simulink model "ES228A_HwTqArbn"
settings: Solver=ode45  StartTime=0.0  StopTime=10.0  RelTol=1e-3
values from neighbouring files (symbols this model uses):
  HWTQSCA_CNT_U08 = DataDict.Constant    [ES228A_HwTqArbn_DataDict.m]
libraries: simulink x9, NexteerUtilities x3
settings DataIOCC: LimitDataPoints=on  SaveFormat=Array  ReturnWorkspaceOutputs=off
settings OptimizationCC: LifeSpan=inf  SimCompilerOptimization=Off
settings DebuggingCC: UnderspecifiedInitializationDetection=Classic  MergeDetectMultiDrivingBlocksExec=none  SolverPrmCheckMsg=warning  FcnCallInpInsideContextMsg=EnableAllAsError  FrameProcessingCompatibilityMsg=warning  SFUnexpectedBacktrackingDiag=warning  SFNoUnconditionalDefaultTransitionDiag=warning
settings HardwareCC: ProdBitPerPointer=32  ProdLargestAtomicFloat=None  ProdIntDivRoundTo=Undefined  ProdEndianess=Unspecified  ProdWordSize=32  ProdHWDeviceType=32-bit Generic
settings ModelReferenceCC: PropagateSignalLabelsOutOfModel=off
settings SFSimCC: SimUseLocalCustomCode=off
settings RTWCC: RTWUseLocalCustomCode=off  RTWCompilerOptimization=Off
settings GRTTargetCC: CodeReplacementLibrary=ANSI_C  GeneratePreprocessorConditionals=Disable all  CPPClassGenCompliant=off

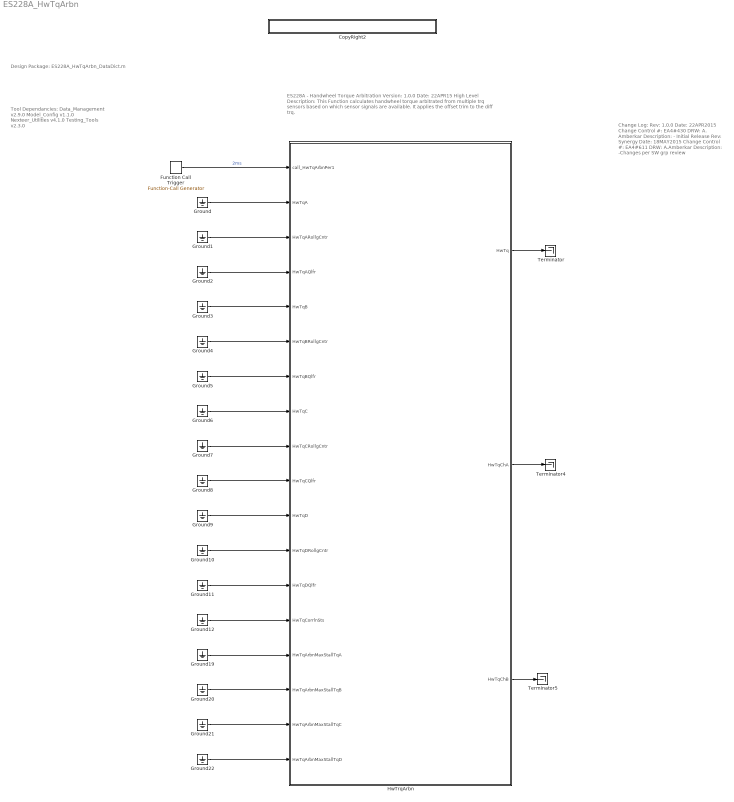
== system ES228A_HwTqArbn ==
  note: Design Package:
      |
      | ES228A_HwTqArbn_DataDict.m
  note: Tool Dependancies:
      |
      | Data_Management v2.9.0
      | Model_Config v1.1.0
      | Nexteer_Utilities v4.1.0
      | Testing_Tools v2.3.0
  note: Change Log:
      |
      | Rev: 1.0.0
      | Date: 22APR2015
      | Change Control #: EA4#430
      | DRW: A. Amberkar
      | Description:
      | - Initial Release
      |
      | Rev: Synergy
      | Date: 18MAY2015
      | Change Control #: EA4#611
      | DRW: A.Amberkar
      | Description:
      | -Changes per SW grp review
  note: ES228A - Handwheel Torque Arbitration
      |
      | Version: 1.0.0
      | Date: 22APR15
      |
      | High Level Description:
      | This Function calculates handwheel torque arbitrated from multiple trq sensors based
      | on which sensor signals are available.  It applies the offset trim to the diff trq.
  CopyRight2 : Subsystem  Description=|  mask(Copyright Information){none=on}
      | Copyright info block.                                               
      |                                                                     
      | Place copyright information at the top of every subsystem in design.
      mask prompts: none "No parameters"
      mask help: Place copyright information at the top of every subsystem in design.
      mask Display:
      | NxtrConf = 'Nexteer Confidential';
      | 
      | sys = bdroot; %handle for the current model ("system")
      | first = get_param(sys,'Created');
      | first = first(end-3:end);  %year is last four digits
      | 
      | last = get_param(sys,'LastModifiedDate');
      | if isempty(last)
      |     last = datestr(now,'yyyy');
      | else
      |     last = last(end-3:end);
      | end
      | 
      | if strcmp(first,last)
      |     fprintf('%s -- Copyright %s Nexteer',NxtrConf,first)
      | else
      |     fprintf('%s -- %s%s- %s Nexteer',NxtrConf,char(169),first,last)
      | end
  Function Call Trigger : simulink/Ports & Subsystems/Function-Call Generator  sample_time=.002  numberOfIterations=1
  Ground{,1..12,19..22} (17 alike) : Ground
  HwTrqArbn : Subsystem
  Terminator : Terminator
  Terminator4 : Terminator
  Terminator5 : Terminator
  wires:
  Function Call Trigger/1 -> HwTrqArbn/1(call_HwTqArbnPer1)  "2ms"
  HwTrqArbn/2(HwTqChA) -> Terminator4/1
  HwTrqArbn/1(HwTq) -> Terminator/1
  Ground1/1 -> HwTrqArbn/3(HwTqARollgCntr)
  Ground3/1 -> HwTrqArbn/5(HwTqB)
  Ground5/1 -> HwTrqArbn/7(HwTqBQlfr)
  Ground9/1 -> HwTrqArbn/11(HwTqD)
  Ground10/1 -> HwTrqArbn/12(HwTqDRollgCntr)
  Ground11/1 -> HwTrqArbn/13(HwTqDQlfr)
  Ground12/1 -> HwTrqArbn/14(HwTqCorrlnSts)
  Ground20/1 -> HwTrqArbn/16(HwTqArbnMaxStallTqB)
  Ground21/1 -> HwTrqArbn/17(HwTqArbnMaxStallTqC)
  Ground22/1 -> HwTrqArbn/18(HwTqArbnMaxStallTqD)
  Ground8/1 -> HwTrqArbn/10(HwTqCQlfr)
  Ground4/1 -> HwTrqArbn/6(HwTqBRollgCntr)
  Ground/1 -> HwTrqArbn/2(HwTqA)
  HwTrqArbn/3(HwTqChB) -> Terminator5/1
  Ground2/1 -> HwTrqArbn/4(HwTqAQlfr)
  Ground19/1 -> HwTrqArbn/15("HwTqArbnMaxStallTqA ")
  Ground7/1 -> HwTrqArbn/9(HwTqCRollgCntr)
  Ground6/1 -> HwTrqArbn/8(HwTqC)

== system ES228A_HwTqArbn/CopyRight2 ==

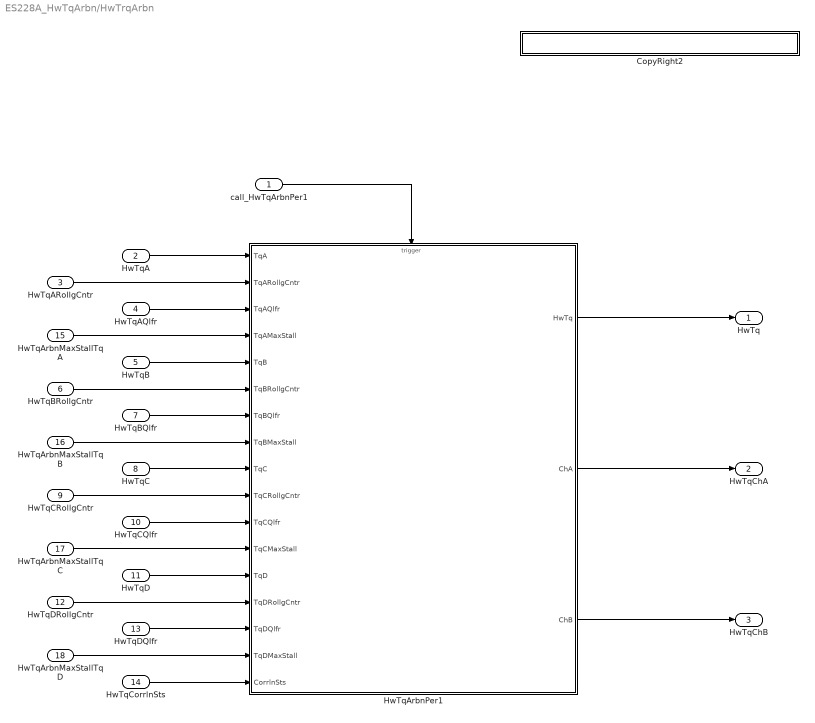
== system ES228A_HwTqArbn/HwTrqArbn ==
  call_HwTqArbnPer1 : Inport
  HwTqA : Inport  Port=2
  HwTqARollgCntr : Inport  Port=3
  HwTqAQlfr : Inport  Port=4
  HwTqB : Inport  Port=5
  HwTqBRollgCntr : Inport  Port=6
  HwTqBQlfr : Inport  Port=7
  HwTqC : Inport  Port=8
  HwTqCRollgCntr : Inport  Port=9
  HwTqCQlfr : Inport  Port=10
  HwTqD : Inport  Port=11
  HwTqDRollgCntr : Inport  Port=12
  HwTqDQlfr : Inport  Port=13
  HwTqCorrlnSts : Inport  Port=14
  "HwTqArbnMaxStallTqA " : Inport  Port=15
  HwTqArbnMaxStallTqB : Inport  Port=16
  HwTqArbnMaxStallTqC : Inport  Port=17
  HwTqArbnMaxStallTqD : Inport  Port=18
  CopyRight2 : Subsystem  Description=|  mask(Copyright Information){none=on}
      | Copyright info block.                                               
      |                                                                     
      | Place copyright information at the top of every subsystem in design.
      mask prompts: none "No parameters"
      mask help: Place copyright information at the top of every subsystem in design.
      mask Display:
      | NxtrConf = 'Nexteer Confidential';
      | 
      | sys = bdroot; %handle for the current model ("system")
      | first = get_param(sys,'Created');
      | first = first(end-3:end);  %year is last four digits
      | 
      | last = get_param(sys,'LastModifiedDate');
      | if isempty(last)
      |     last = datestr(now,'yyyy');
      | else
      |     last = last(end-3:end);
      | end
      | 
      | if strcmp(first,last)
      |     fprintf('%s -- Copyright %s Nexteer',NxtrConf,first)
      | else
      |     fprintf('%s -- %s%s- %s Nexteer',NxtrConf,char(169),first,last)
      | end
  HwTqArbnPer1 : Subsystem  RequirementInfo="{'linktype_rmi_doors' '0000c476 (/ESG Group/FDD Module Requirements/EA4 Specific/ES228A_HwTqArbn)' '#ES228A_85' 'true' 'REQ:  ES228A_85' '' } %GIDa_343f2210_b87e_41f4_8880_c295a6f80a3f"  TreatAsAtomicUnit=on
  HwTq : Outport
  HwTqChA : Outport  Port=2
  HwTqChB : Outport  Port=3
  wires:
  call_HwTqArbnPer1/1 -> HwTqArbnPer1/Trigger
  HwTqARollgCntr/1 -> HwTqArbnPer1/2(TqARollgCntr)
  HwTqAQlfr/1 -> HwTqArbnPer1/3(TqAQlfr)
  HwTqBRollgCntr/1 -> HwTqArbnPer1/6(TqBRollgCntr)
  HwTqBQlfr/1 -> HwTqArbnPer1/7(TqBQlfr)
  HwTqCRollgCntr/1 -> HwTqArbnPer1/10(TqCRollgCntr)
  HwTqCQlfr/1 -> HwTqArbnPer1/11(TqCQlfr)
  HwTqDRollgCntr/1 -> HwTqArbnPer1/14(TqDRollgCntr)
  HwTqDQlfr/1 -> HwTqArbnPer1/15(TqDQlfr)
  "HwTqArbnMaxStallTqA "/1 -> HwTqArbnPer1/4(TqAMaxStall)
  HwTqCorrlnSts/1 -> HwTqArbnPer1/17(CorrlnSts)
  HwTqArbnMaxStallTqC/1 -> HwTqArbnPer1/12(TqCMaxStall)
  HwTqArbnMaxStallTqD/1 -> HwTqArbnPer1/16(TqDMaxStall)
  HwTqA/1 -> HwTqArbnPer1/1(TqA)
  HwTqB/1 -> HwTqArbnPer1/5(TqB)
  HwTqArbnMaxStallTqB/1 -> HwTqArbnPer1/8(TqBMaxStall)
  HwTqC/1 -> HwTqArbnPer1/9(TqC)
  HwTqD/1 -> HwTqArbnPer1/13(TqD)
  HwTqArbnPer1/1(HwTq) -> HwTq/1
  HwTqArbnPer1/2(ChA) -> HwTqChA/1
  HwTqArbnPer1/3(ChB) -> HwTqChB/1

== system ES228A_HwTqArbn/HwTrqArbn/CopyRight2 ==

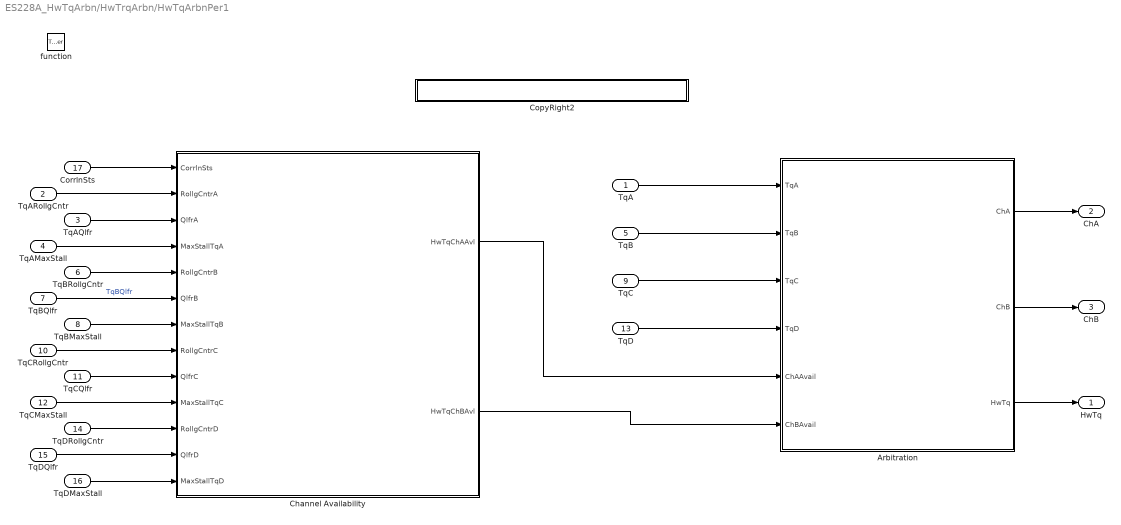
== system ES228A_HwTqArbn/HwTrqArbn/HwTqArbnPer1 ==
  TqA : Inport
  TqARollgCntr : Inport  Port=2
  TqAQlfr : Inport  Port=3
  TqAMaxStall : Inport  Port=4
  TqB : Inport  Port=5
  TqBRollgCntr : Inport  Port=6
  TqBQlfr : Inport  Port=7
  TqBMaxStall : Inport  Port=8
  TqC : Inport  Port=9
  TqCRollgCntr : Inport  Port=10
  TqCQlfr : Inport  Port=11
  TqCMaxStall : Inport  Port=12
  TqD : Inport  Port=13
  TqDRollgCntr : Inport  Port=14
  TqDQlfr : Inport  Port=15
  TqDMaxStall : Inport  Port=16
  CorrlnSts : Inport  Port=17
  function : TriggerPort  TriggerType=function-call
  Arbitration : Subsystem  RequirementInfo="{'linktype_rmi_doors' '0000c476 (/ESG Group/FDD Module Requirements/EA4 Specific/ES228A_HwTqArbn)' '#ES228A_128' 'true' 'REQ:  ES228A_128' '' ; 'linktype_rmi_doors' '0000c476 (/ESG Group/FDD Module Requirements/EA4 Specific/ES228A_HwTqArbn)' '#ES228A_98' 'true' 'REQ:  ES228A_98' '' } %GIDa_5e475dce_6d1a_4377_b1f7_ac9d58e1cf5d"
  Channel Availability : Subsystem
  CopyRight2 : Subsystem  Description=|  mask(Copyright Information){none=on}
      | Copyright info block.                                               
      |                                                                     
      | Place copyright information at the top of every subsystem in design.
      mask prompts: none "No parameters"
      mask help: Place copyright information at the top of every subsystem in design.
      mask Display:
      | NxtrConf = 'Nexteer Confidential';
      | 
      | sys = bdroot; %handle for the current model ("system")
      | first = get_param(sys,'Created');
      | first = first(end-3:end);  %year is last four digits
      | 
      | last = get_param(sys,'LastModifiedDate');
      | if isempty(last)
      |     last = datestr(now,'yyyy');
      | else
      |     last = last(end-3:end);
      | end
      | 
      | if strcmp(first,last)
      |     fprintf('%s -- Copyright %s Nexteer',NxtrConf,first)
      | else
      |     fprintf('%s -- %s%s- %s Nexteer',NxtrConf,char(169),first,last)
      | end
  HwTq : Outport
  ChA : Outport  Port=2
  ChB : Outport  Port=3
  wires:
  CorrlnSts/1 -> Channel Availability/1(CorrlnSts)
  TqAQlfr/1 -> Channel Availability/3(QlfrA)
  TqAMaxStall/1 -> Channel Availability/4(MaxStallTqA)
  TqBRollgCntr/1 -> Channel Availability/5(RollgCntrB)
  TqBQlfr/1 -> Channel Availability/6(QlfrB)  "TqBQlfr"
  TqBMaxStall/1 -> Channel Availability/7(MaxStallTqB)
  TqCRollgCntr/1 -> Channel Availability/8(RollgCntrC)
  TqCQlfr/1 -> Channel Availability/9(QlfrC)
  TqCMaxStall/1 -> Channel Availability/10(MaxStallTqC)
  TqDRollgCntr/1 -> Channel Availability/11(RollgCntrD)
  TqDQlfr/1 -> Channel Availability/12(QlfrD)
  TqDMaxStall/1 -> Channel Availability/13(MaxStallTqD)
  TqARollgCntr/1 -> Channel Availability/2(RollgCntrA)
  TqA/1 -> Arbitration/1(TqA)
  TqB/1 -> Arbitration/2(TqB)
  TqC/1 -> Arbitration/3(TqC)
  TqD/1 -> Arbitration/4(TqD)
  Channel Availability/1(HwTqChAAvl) -> Arbitration/5(ChAAvail)
  Channel Availability/2(HwTqChBAvl) -> Arbitration/6(ChBAvail)
  Arbitration/3(HwTq) -> HwTq/1
  Arbitration/2(ChB) -> ChB/1
  Arbitration/1(ChA) -> ChA/1

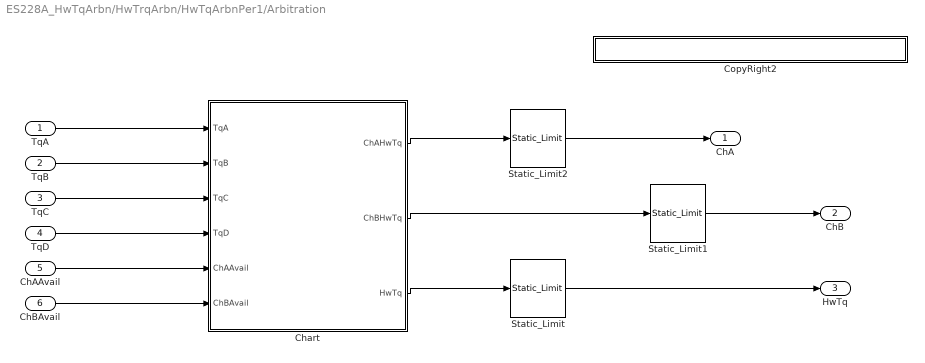
== system ES228A_HwTqArbn/HwTrqArbn/HwTqArbnPer1/Arbitration ==
  TqA : Inport
  TqB : Inport  Port=2
  TqC : Inport  Port=3
  TqD : Inport  Port=4
  ChAAvail : Inport  Port=5
  ChBAvail : Inport  Port=6
  Chart : Stateflow chart  RequirementInfo="{'linktype_rmi_doors' '0000c476 (/ESG Group/FDD Module Requirements/EA4 Specific/ES228A_HwTqArbn)' '#ES228A_83' 'true' 'REQ:  ES228A_83' '' } %GIDa_6d64dbbd_6a35_4759_a8d5_33867a77d9f5"  TreatAsAtomicUnit=on
  CopyRight2 : Subsystem  Description=|  mask(Copyright Information){none=on}
      | Copyright info block.                                               
      |                                                                     
      | Place copyright information at the top of every subsystem in design.
      mask prompts: none "No parameters"
      mask help: Place copyright information at the top of every subsystem in design.
      mask Display:
      | NxtrConf = 'Nexteer Confidential';
      | 
      | sys = bdroot; %handle for the current model ("system")
      | first = get_param(sys,'Created');
      | first = first(end-3:end);  %year is last four digits
      | 
      | last = get_param(sys,'LastModifiedDate');
      | if isempty(last)
      |     last = datestr(now,'yyyy');
      | else
      |     last = last(end-3:end);
      | end
      | 
      | if strcmp(first,last)
      |     fprintf('%s -- Copyright %s Nexteer',NxtrConf,first)
      | else
      |     fprintf('%s -- %s%s- %s Nexteer',NxtrConf,char(169),first,last)
      | end
  Static_Limit : NexteerUtilities/Static_Limit  uprlim=HWTQMAXLIM_HWNWTMTR_F32  lwrlim=HWTQMINLIM_HWNWTMTR_F32
      settings: AttributesFormatString=|
      | Upper Limit:%<uprlim>
      | Lower Limit:%<lwrlim>
  Static_Limit1 : NexteerUtilities/Static_Limit  uprlim=HWTQMAXLIM_HWNWTMTR_F32  lwrlim=HWTQMINLIM_HWNWTMTR_F32
      settings: AttributesFormatString=|
      | Upper Limit:%<uprlim>
      | Lower Limit:%<lwrlim>
  Static_Limit2 : NexteerUtilities/Static_Limit  uprlim=HWTQMAXLIM_HWNWTMTR_F32  lwrlim=HWTQMINLIM_HWNWTMTR_F32
      settings: AttributesFormatString=|
      | Upper Limit:%<uprlim>
      | Lower Limit:%<lwrlim>
  ChA : Outport
  ChB : Outport  Port=2
  HwTq : Outport  Port=3
  wires:
  TqA/1 -> Chart/1(TqA)
  TqB/1 -> Chart/2(TqB)
  TqC/1 -> Chart/3(TqC)
  TqD/1 -> Chart/4(TqD)
  ChAAvail/1 -> Chart/5(ChAAvail)
  ChBAvail/1 -> Chart/6(ChBAvail)
  Chart/1(ChAHwTq) -> Static_Limit2/1
  Chart/2(ChBHwTq) -> Static_Limit1/1
  Chart/3(HwTq) -> Static_Limit/1
  Static_Limit/1 -> HwTq/1
  Static_Limit1/1 -> ChB/1
  Static_Limit2/1 -> ChA/1

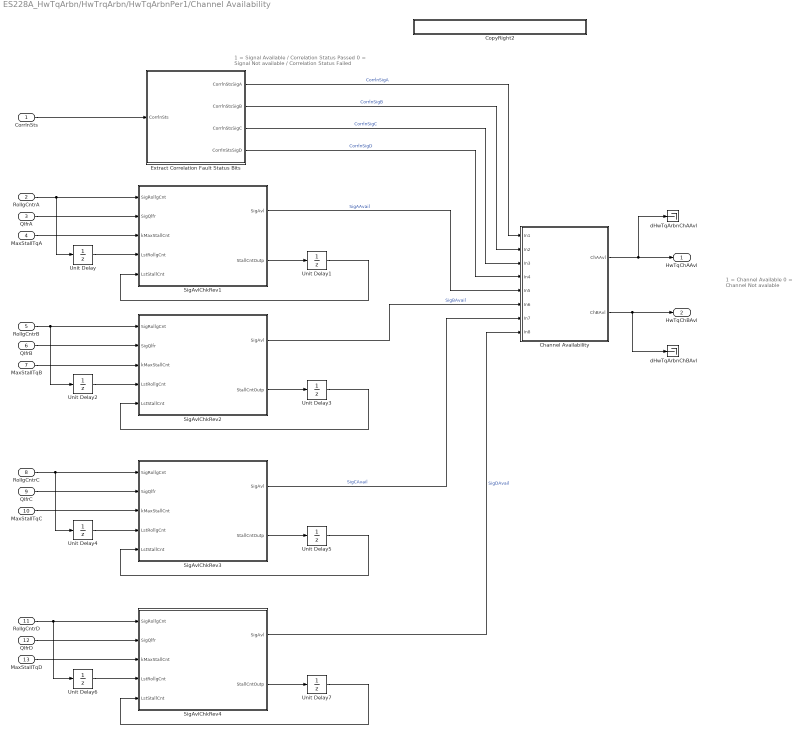
== system ES228A_HwTqArbn/HwTrqArbn/HwTqArbnPer1/Channel Availability ==
  note: 1 = Channel Available
      | 0 = Channel Not avalable
  note: 1 = Signal Available / Correlation Status Passed
      | 0 = Signal Not available / Correlation Status Failed
  CorrlnSts : Inport
  RollgCntrA : Inport  Port=2
  QlfrA : Inport  Port=3
  MaxStallTqA : Inport  Port=4
  RollgCntrB : Inport  Port=5
  QlfrB : Inport  Port=6
  MaxStallTqB : Inport  Port=7
  RollgCntrC : Inport  Port=8
  QlfrC : Inport  Port=9
  MaxStallTqC : Inport  Port=10
  RollgCntrD : Inport  Port=11
  QlfrD : Inport  Port=12
  MaxStallTqD : Inport  Port=13
  Channel Availability : Subsystem  RequirementInfo="{'linktype_rmi_doors' '0000c476 (/ESG Group/FDD Module Requirements/EA4 Specific/ES228A_HwTqArbn)' '#ES228A_129' 'true' 'REQ:  ES228A_129' '' ; 'linktype_rmi_doors' '0000c476 (/ESG Group/FDD Module Requirements/EA4 Specific/ES228A_HwTqArbn)' '#ES228A_91' 'true' 'REQ:  ES228A_91' '' } %GIDa_746ca483_b495_4e00_a250_9b34cc012507"
  CopyRight2 : Subsystem  Description=|  mask(Copyright Information){none=on}
      | Copyright info block.                                               
      |                                                                     
      | Place copyright information at the top of every subsystem in design.
      mask prompts: none "No parameters"
      mask help: Place copyright information at the top of every subsystem in design.
      mask Display:
      | NxtrConf = 'Nexteer Confidential';
      | 
      | sys = bdroot; %handle for the current model ("system")
      | first = get_param(sys,'Created');
      | first = first(end-3:end);  %year is last four digits
      | 
      | last = get_param(sys,'LastModifiedDate');
      | if isempty(last)
      |     last = datestr(now,'yyyy');
      | else
      |     last = last(end-3:end);
      | end
      | 
      | if strcmp(first,last)
      |     fprintf('%s -- Copyright %s Nexteer',NxtrConf,first)
      | else
      |     fprintf('%s -- %s%s- %s Nexteer',NxtrConf,char(169),first,last)
      | end
  Extract Correlation Fault Status Bits : Subsystem  RequirementInfo="{'linktype_rmi_doors' '0000c476 (/ESG Group/FDD Module Requirements/EA4 Specific/ES228A_HwTqArbn)' '#ES228A_129' 'true' 'REQ:  ES228A_129' '' } %GIDa_e59e4d92_3888_4f3c_9500_97095e00bcfc"
  SigAvlChkRev1 : Stateflow chart  RequirementInfo="{'linktype_rmi_doors' '0000c476 (/ESG Group/FDD Module Requirements/EA4 Specific/ES228A_HwTqArbn)' '#ES228A_91' 'true' 'REQ:  ES228A_91' '' } %GIDa_e4c178c2_f8a5_42cf_ac9f_6f496b5237f8"  TreatAsAtomicUnit=on
  SigAvlChkRev2 : Stateflow chart  RequirementInfo="{'linktype_rmi_doors' '0000c476 (/ESG Group/FDD Module Requirements/EA4 Specific/ES228A_HwTqArbn)' '#ES228A_91' 'true' 'REQ:  ES228A_91' '' } %GIDa_b0676f02_3d97_45d5_aa8a_49c82560c074"  TreatAsAtomicUnit=on
  SigAvlChkRev3 : Stateflow chart  RequirementInfo="{'linktype_rmi_doors' '0000c476 (/ESG Group/FDD Module Requirements/EA4 Specific/ES228A_HwTqArbn)' '#ES228A_91' 'true' 'REQ:  ES228A_91' '' } %GIDa_99c29bb1_dae8_491f_835b_8ea19b5dfde5"  TreatAsAtomicUnit=on
  SigAvlChkRev4 : Stateflow chart  RequirementInfo="{'linktype_rmi_doors' '0000c476 (/ESG Group/FDD Module Requirements/EA4 Specific/ES228A_HwTqArbn)' '#ES228A_91' 'true' 'REQ:  ES228A_91' '' } %GIDa_0917a9fe_5043_4981_abf9_3e4589195506"  TreatAsAtomicUnit=on
  Unit Delay : UnitDelay  SampleTime=-1  StateName=HwTqArbnTqARollgCntrPrev  StateMustResolveToSignalObject=on
      settings: AttributesFormatString=|
      | State Variable:
      | %<StateName>
  Unit Delay1 : UnitDelay  SampleTime=-1  StateName=HwTqArbnTqAStallCntrPrev  StateMustResolveToSignalObject=on
      settings: AttributesFormatString=|
      | State Variable:
      | %<StateName>
  Unit Delay2 : UnitDelay  SampleTime=-1  StateName=HwTqArbnTqBRollgCntrPrev  StateMustResolveToSignalObject=on
      settings: AttributesFormatString=|
      | State Variable:
      | %<StateName>
  Unit Delay3 : UnitDelay  SampleTime=-1  StateName=HwTqArbnTqBStallCntrPrev  StateMustResolveToSignalObject=on
      settings: AttributesFormatString=|
      | State Variable:
      | %<StateName>
  Unit Delay4 : UnitDelay  SampleTime=-1  StateName=HwTqArbnTqCRollgCntrPrev  StateMustResolveToSignalObject=on
      settings: AttributesFormatString=|
      | State Variable:
      | %<StateName>
  Unit Delay5 : UnitDelay  SampleTime=-1  StateName=HwTqArbnTqCStallCntrPrev  StateMustResolveToSignalObject=on
      settings: AttributesFormatString=|
      | State Variable:
      | %<StateName>
  Unit Delay6 : UnitDelay  SampleTime=-1  StateName=HwTqArbnTqDRollgCntrPrev  StateMustResolveToSignalObject=on
      settings: AttributesFormatString=|
      | State Variable:
      | %<StateName>
  Unit Delay7 : UnitDelay  SampleTime=-1  StateName=HwTqArbnTqDStallCntrPrev  StateMustResolveToSignalObject=on
      settings: AttributesFormatString=|
      | State Variable:
      | %<StateName>
  "dHwTqArbnChAAvl " : Terminator
  "dHwTqArbnChBAvl " : Terminator
  HwTqChAAvl : Outport
  HwTqChBAvl : Outport  Port=2
  wires:
  CorrlnSts/1 -> Extract Correlation Fault Status Bits/1(CorrlnSts)
  Extract Correlation Fault Status Bits/1(CorrlnStsSigA) -> Channel Availability/1(In1)  "CorrlnSigA"
  Extract Correlation Fault Status Bits/2(CorrlnStsSigB) -> Channel Availability/2(In2)  "CorrlnSigB"
  Extract Correlation Fault Status Bits/3(CorrlnStsSigC) -> Channel Availability/3(In3)  "CorrlnSigC"
  Extract Correlation Fault Status Bits/4(CorrlnStsSigD) -> Channel Availability/4(In4)  "CorrlnSigD"
  SigAvlChkRev1/1(SigAvl) -> Channel Availability/5(In5)  "SigAAvail"
  SigAvlChkRev2/1(SigAvl) -> Channel Availability/6(In6)  "SigBAvail"
  SigAvlChkRev3/1(SigAvl) -> Channel Availability/7(In7)  "SigCAvail"
  SigAvlChkRev4/1(SigAvl) -> Channel Availability/8(In8)  "SigDAvail"
  Channel Availability/1(ChAAvl) -> "dHwTqArbnChAAvl "/1, HwTqChAAvl/1
  Channel Availability/2(ChBAvl) -> "dHwTqArbnChBAvl "/1, HwTqChBAvl/1
  RollgCntrA/1 -> Unit Delay/1, SigAvlChkRev1/1(SigRollgCnt)
  QlfrA/1 -> SigAvlChkRev1/2(SigQlfr)
  MaxStallTqA/1 -> SigAvlChkRev1/3(kMaxStallCnt)
  RollgCntrB/1 -> Unit Delay2/1, SigAvlChkRev2/1(SigRollgCnt)
  QlfrB/1 -> SigAvlChkRev2/2(SigQlfr)
  MaxStallTqB/1 -> SigAvlChkRev2/3(kMaxStallCnt)
  RollgCntrC/1 -> Unit Delay4/1, SigAvlChkRev3/1(SigRollgCnt)
  QlfrC/1 -> SigAvlChkRev3/2(SigQlfr)
  MaxStallTqC/1 -> SigAvlChkRev3/3(kMaxStallCnt)
  RollgCntrD/1 -> Unit Delay6/1, SigAvlChkRev4/1(SigRollgCnt)
  QlfrD/1 -> SigAvlChkRev4/2(SigQlfr)
  MaxStallTqD/1 -> SigAvlChkRev4/3(kMaxStallCnt)
  Unit Delay/1 -> SigAvlChkRev1/4(LstRollgCnt)
  SigAvlChkRev1/2(StallCntOutp) -> Unit Delay1/1
  Unit Delay1/1 -> SigAvlChkRev1/5(LstStallCnt)
  Unit Delay2/1 -> SigAvlChkRev2/4(LstRollgCnt)
  SigAvlChkRev2/2(StallCntOutp) -> Unit Delay3/1
  Unit Delay3/1 -> SigAvlChkRev2/5(LstStallCnt)
  Unit Delay4/1 -> SigAvlChkRev3/4(LstRollgCnt)
  SigAvlChkRev3/2(StallCntOutp) -> Unit Delay5/1
  Unit Delay5/1 -> SigAvlChkRev3/5(LstStallCnt)
  Unit Delay6/1 -> SigAvlChkRev4/4(LstRollgCnt)
  SigAvlChkRev4/2(StallCntOutp) -> Unit Delay7/1
  Unit Delay7/1 -> SigAvlChkRev4/5(LstStallCnt)

== system ES228A_HwTqArbn/HwTrqArbn/HwTqArbnPer1/CopyRight2 ==

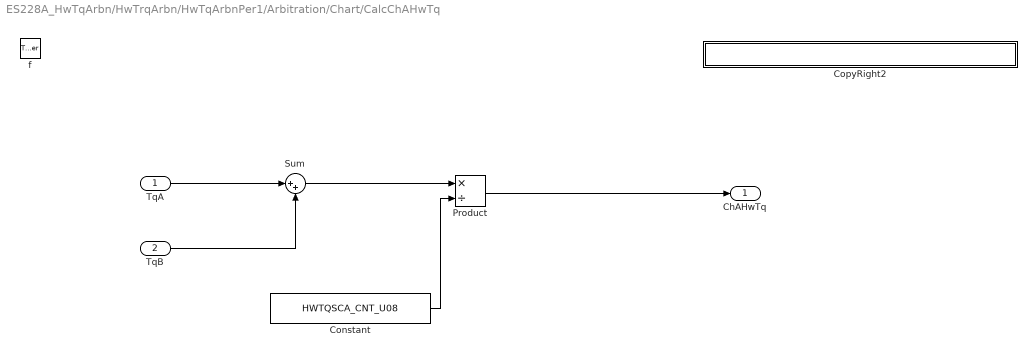
== system ES228A_HwTqArbn/HwTrqArbn/HwTqArbnPer1/Arbitration/Chart/CalcChAHwTq ==
  TqA : Inport
  TqB : Inport  Port=2
  f : TriggerPort  TriggerType=function-call
      settings: CopyFcn=Stateflow.SLINSF.SimulinkMan.removeBlockPreDeleteFcn  PreDeleteFcn=Stateflow.SLINSF.SimulinkMan.unsafePredeleteFcn
  Constant : Constant  Value=HWTQSCA_CNT_U08
  CopyRight2 : Subsystem  Description=|  mask(Copyright Information){none=on}
      | Copyright info block.                                               
      |                                                                     
      | Place copyright information at the top of every subsystem in design.
      mask prompts: none "No parameters"
      mask help: Place copyright information at the top of every subsystem in design.
      mask Display:
      | NxtrConf = 'Nexteer Confidential';
      | 
      | sys = bdroot; %handle for the current model ("system")
      | first = get_param(sys,'Created');
      | first = first(end-3:end);  %year is last four digits
      | 
      | last = get_param(sys,'LastModifiedDate');
      | if isempty(last)
      |     last = datestr(now,'yyyy');
      | else
      |     last = last(end-3:end);
      | end
      | 
      | if strcmp(first,last)
      |     fprintf('%s -- Copyright %s Nexteer',NxtrConf,first)
      | else
      |     fprintf('%s -- %s%s- %s Nexteer',NxtrConf,char(169),first,last)
      | end
  Product : Product  Inputs=*/
  Sum : Sum  Inputs=|++
  ChAHwTq : Outport
  wires:
  TqA/1 -> Sum/1
  TqB/1 -> Sum/2
  Sum/1 -> Product/1
  Constant/1 -> Product/2
  Product/1 -> ChAHwTq/1

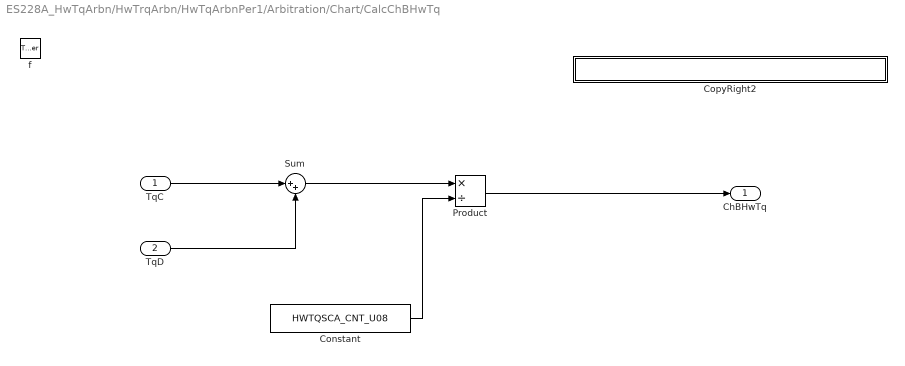
== system ES228A_HwTqArbn/HwTrqArbn/HwTqArbnPer1/Arbitration/Chart/CalcChBHwTq ==
  TqC : Inport
  TqD : Inport  Port=2
  f : TriggerPort  TriggerType=function-call
      settings: CopyFcn=Stateflow.SLINSF.SimulinkMan.removeBlockPreDeleteFcn  PreDeleteFcn=Stateflow.SLINSF.SimulinkMan.unsafePredeleteFcn
  Constant : Constant  Value=HWTQSCA_CNT_U08
  CopyRight2 : Subsystem  Description=|  mask(Copyright Information){none=on}
      | Copyright info block.                                               
      |                                                                     
      | Place copyright information at the top of every subsystem in design.
      mask prompts: none "No parameters"
      mask help: Place copyright information at the top of every subsystem in design.
      mask Display:
      | NxtrConf = 'Nexteer Confidential';
      | 
      | sys = bdroot; %handle for the current model ("system")
      | first = get_param(sys,'Created');
      | first = first(end-3:end);  %year is last four digits
      | 
      | last = get_param(sys,'LastModifiedDate');
      | if isempty(last)
      |     last = datestr(now,'yyyy');
      | else
      |     last = last(end-3:end);
      | end
      | 
      | if strcmp(first,last)
      |     fprintf('%s -- Copyright %s Nexteer',NxtrConf,first)
      | else
      |     fprintf('%s -- %s%s- %s Nexteer',NxtrConf,char(169),first,last)
      | end
  Product : Product  Inputs=*/
  Sum : Sum  Inputs=|++
  ChBHwTq : Outport
  wires:
  TqC/1 -> Sum/1
  TqD/1 -> Sum/2
  Sum/1 -> Product/1
  Constant/1 -> Product/2
  Product/1 -> ChBHwTq/1

== system ES228A_HwTqArbn/HwTrqArbn/HwTqArbnPer1/Arbitration/CopyRight2 ==

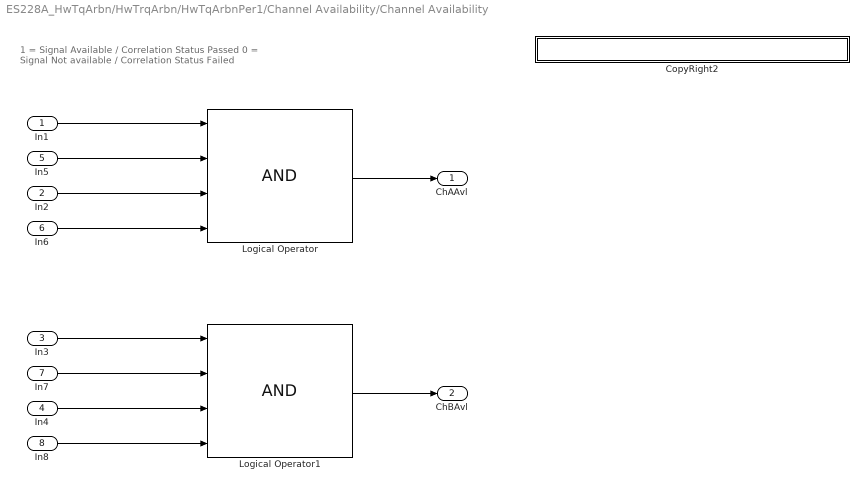
== system ES228A_HwTqArbn/HwTrqArbn/HwTqArbnPer1/Channel Availability/Channel Availability ==
  note: 1 = Signal Available / Correlation Status Passed
      | 0 = Signal Not available / Correlation Status Failed
  In1 : Inport
  In2 : Inport  Port=2
  In3 : Inport  Port=3
  In4 : Inport  Port=4
  In5 : Inport  Port=5
  In6 : Inport  Port=6
  In7 : Inport  Port=7
  In8 : Inport  Port=8
  CopyRight2 : Subsystem  Description=|  mask(Copyright Information){none=on}
      | Copyright info block.                                               
      |                                                                     
      | Place copyright information at the top of every subsystem in design.
      mask prompts: none "No parameters"
      mask help: Place copyright information at the top of every subsystem in design.
      mask Display:
      | NxtrConf = 'Nexteer Confidential';
      | 
      | sys = bdroot; %handle for the current model ("system")
      | first = get_param(sys,'Created');
      | first = first(end-3:end);  %year is last four digits
      | 
      | last = get_param(sys,'LastModifiedDate');
      | if isempty(last)
      |     last = datestr(now,'yyyy');
      | else
      |     last = last(end-3:end);
      | end
      | 
      | if strcmp(first,last)
      |     fprintf('%s -- Copyright %s Nexteer',NxtrConf,first)
      | else
      |     fprintf('%s -- %s%s- %s Nexteer',NxtrConf,char(169),first,last)
      | end
  Logical Operator : Logic  Inputs=4  AllPortsSameDT=off  OutDataTypeStr=boolean
  Logical Operator1 : Logic  Inputs=4  AllPortsSameDT=off  OutDataTypeStr=boolean
  ChAAvl : Outport
  ChBAvl : Outport  Port=2
  wires:
  In1/1 -> Logical Operator/1
  In5/1 -> Logical Operator/2
  In2/1 -> Logical Operator/3
  In6/1 -> Logical Operator/4
  Logical Operator/1 -> ChAAvl/1
  In3/1 -> Logical Operator1/1
  In7/1 -> Logical Operator1/2
  In4/1 -> Logical Operator1/3
  In8/1 -> Logical Operator1/4
  Logical Operator1/1 -> ChBAvl/1

== system ES228A_HwTqArbn/HwTrqArbn/HwTqArbnPer1/Channel Availability/CopyRight2 ==

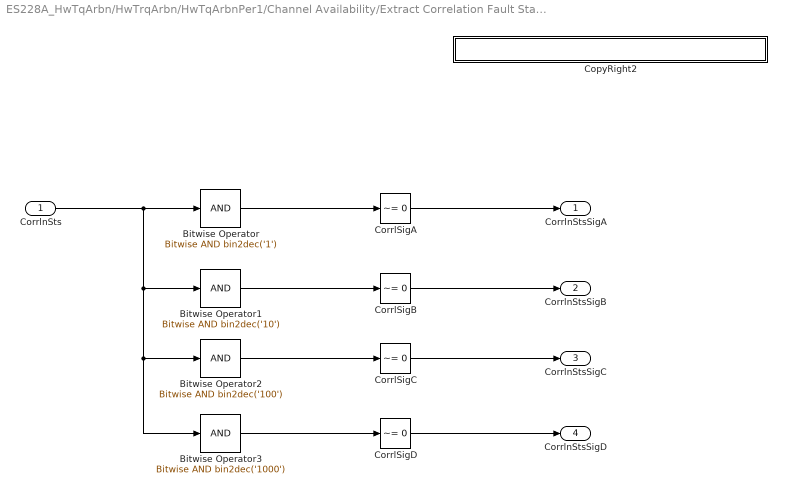
== system ES228A_HwTqArbn/HwTrqArbn/HwTqArbnPer1/Channel Availability/Extract Correlation Fault Status Bits ==
  CorrlnSts : Inport
  Bitwise Operator : simulink/Logic and Bit Operations/Bitwise Operator  logicop=AND  UseBitMask=on  BitMask=bin2dec('1')  BitMaskRealWorld=Stored Integer
  Bitwise Operator1 : simulink/Logic and Bit Operations/Bitwise Operator  logicop=AND  UseBitMask=on  BitMask=bin2dec('10')  BitMaskRealWorld=Stored Integer
  Bitwise Operator2 : simulink/Logic and Bit Operations/Bitwise Operator  logicop=AND  UseBitMask=on  BitMask=bin2dec('100')  BitMaskRealWorld=Stored Integer
  Bitwise Operator3 : simulink/Logic and Bit Operations/Bitwise Operator  logicop=AND  UseBitMask=on  BitMask=bin2dec('1000')  BitMaskRealWorld=Stored Integer
  CopyRight2 : Subsystem  Description=|  mask(Copyright Information){none=on}
      | Copyright info block.                                               
      |                                                                     
      | Place copyright information at the top of every subsystem in design.
      mask prompts: none "No parameters"
      mask help: Place copyright information at the top of every subsystem in design.
      mask Display:
      | NxtrConf = 'Nexteer Confidential';
      | 
      | sys = bdroot; %handle for the current model ("system")
      | first = get_param(sys,'Created');
      | first = first(end-3:end);  %year is last four digits
      | 
      | last = get_param(sys,'LastModifiedDate');
      | if isempty(last)
      |     last = datestr(now,'yyyy');
      | else
      |     last = last(end-3:end);
      | end
      | 
      | if strcmp(first,last)
      |     fprintf('%s -- Copyright %s Nexteer',NxtrConf,first)
      | else
      |     fprintf('%s -- %s%s- %s Nexteer',NxtrConf,char(169),first,last)
      | end
  CorrlSigA : simulink/Logic and Bit Operations/Compare To Zero  relop=~=  OutDataTypeStr=boolean
  CorrlSigB : simulink/Logic and Bit Operations/Compare To Zero  relop=~=  OutDataTypeStr=boolean
  CorrlSigC : simulink/Logic and Bit Operations/Compare To Zero  relop=~=  OutDataTypeStr=boolean
  CorrlSigD : simulink/Logic and Bit Operations/Compare To Zero  relop=~=  OutDataTypeStr=boolean
  CorrlnStsSigA : Outport
  CorrlnStsSigB : Outport  Port=2
  CorrlnStsSigC : Outport  Port=3
  CorrlnStsSigD : Outport  Port=4
  wires:
  Bitwise Operator/1 -> CorrlSigA/1
  Bitwise Operator1/1 -> CorrlSigB/1
  Bitwise Operator2/1 -> CorrlSigC/1
  Bitwise Operator3/1 -> CorrlSigD/1
  CorrlSigA/1 -> CorrlnStsSigA/1
  CorrlSigB/1 -> CorrlnStsSigB/1
  CorrlSigC/1 -> CorrlnStsSigC/1
  CorrlSigD/1 -> CorrlnStsSigD/1
  CorrlnSts/1 -> Bitwise Operator/1, Bitwise Operator1/1, Bitwise Operator3/1, Bitwise Operator2/1

== system ES228A_HwTqArbn/HwTrqArbn/HwTqArbnPer1/Arbitration/Chart/CalcChAHwTq/CopyRight2 ==

== system ES228A_HwTqArbn/HwTrqArbn/HwTqArbnPer1/Arbitration/Chart/CalcChBHwTq/CopyRight2 ==

== system ES228A_HwTqArbn/HwTrqArbn/HwTqArbnPer1/Channel Availability/Channel Availability/CopyRight2 ==

== system ES228A_HwTqArbn/HwTrqArbn/HwTqArbnPer1/Channel Availability/Extract Correlation Fault Status Bits/CopyRight2 ==

== stateflow chart ES228A_HwTqArbn/HwTrqArbn/HwTqArbnPer1/Arbitration/Chart ==
  state ChAHwTq = CalcChAHwTq(TqA,TqB) [function]
  state ChBHwTq = CalcChBHwTq(TqC,TqD) [function]
  note: Update/write the module output signals ChAHwTq , ChBHwTq and HwTq only when they are available or calculated in the model
  (default) -> (junction 37) : /* Both channels */
  (junction 37) -> (junction 36) [order 1] : [ChAAvail == 1 && ChBAvail == 1]
  (junction 36) -> (junction 35) : {ChAHwTq = CalcChAHwTq(TqA,TqB);
      | ChBHwTq = CalcChBHwTq(TqC,TqD);
      | HwTq = (ChAHwTq + ChBHwTq) / 2;
      | }
  (junction 37) -> (junction 45) [order 2]
  (junction 45) -> (junction 49) : /* Only Ch1 */
  (junction 49) -> (junction 48) [order 1] : [ChAAvail == 1]
  (junction 48) -> (junction 47) : {ChAHwTq = CalcChAHwTq(TqA,TqB);
      | HwTq = ChAHwTq;
      | }
  (junction 35) -> (junction 34)
  (junction 49) -> (junction 50) [order 2]
  (junction 50) -> (junction 57)
  (junction 47) -> (junction 34)
  (junction 57) -> (junction 61) : /* Only Ch2 */
  (junction 61) -> (junction 60) [order 1] : [ChBAvail == 1]
  (junction 61) -> (junction 62) [order 2]
  (junction 60) -> (junction 59) : {ChBHwTq = CalcChBHwTq(TqC,TqD);
      | HwTq = ChBHwTq;
      | }
  (junction 59) -> (junction 34)
  (junction 62) -> (junction 34)
  data: TqA function_input; TqB function_input; ChAHwTq function_output; TqC function_input; TqD function_input; ChBHwTq function_output; TqA input double; TqB input; TqC input; TqD input; ChAAvail input; ChBAvail input; ChAHwTq output; ChBHwTq output; HwTq output double

== stateflow chart ES228A_HwTqArbn/HwTrqArbn/HwTqArbnPer1/Channel Availability/SigAvlChkRev1 ==
  note: SigAvl
      | False = 0
      | Pass = 1
  note: SigQlfr
      | 0 = No Result
      | 1 = Pass
      | 2 = Fail
  (default) -> (junction 2)
  (junction 2) -> (junction 4) [order 1] : [SigRollgCnt ==LstRollgCnt]
  (junction 4) -> (junction 7) [order 2] : {
      | StallCntOutp = LstStallCnt +1;
      | }
  (junction 2) -> (junction 3) [order 2]
  (junction 4) -> (junction 7) [order 1] : [LstStallCnt == 255]
      | {
      | StallCntOutp = 255;
      | }
  (junction 3) -> (junction 7) : {
      | StallCntOutp = 0;
      | }
  (junction 7) -> (junction 10)
  (junction 10) -> (junction 12) [order 1] : [StallCntOutp >=kMaxStallCnt]
  (junction 10) -> (junction 14) [order 2]
  (junction 12) -> (junction 17)
  (junction 14) -> (junction 17) [order 2]
  (junction 14) -> (junction 16) [order 1] : [SigQlfr<2]
  (junction 17) -> (junction 29) : {
      | SigAvl =0;
      | }
  (junction 16) -> (junction 29) : {
      | SigAvl = 1;
      | }
  data: SigRollgCnt input; SigQlfr input; kMaxStallCnt input; SigAvl output uint8; LstRollgCnt input uint8; LstStallCnt input uint8; StallCntOutp output uint8

== stateflow chart ES228A_HwTqArbn/HwTrqArbn/HwTqArbnPer1/Channel Availability/SigAvlChkRev2 ==
  note: SigAvl
      | False = 0
      | Pass = 1
  note: SigQlfr
      | 0 = No Result
      | 1 = Pass
      | 2 = Fail
  (default) -> (junction 2)
  (junction 2) -> (junction 4) [order 1] : [SigRollgCnt ==LstRollgCnt]
  (junction 4) -> (junction 7) [order 2] : {
      | StallCntOutp = LstStallCnt +1;
      | }
  (junction 2) -> (junction 3) [order 2]
  (junction 4) -> (junction 7) [order 1] : [LstStallCnt == 255]
      | {
      | StallCntOutp = 255;
      | }
  (junction 3) -> (junction 7) : {
      | StallCntOutp = 0;
      | }
  (junction 7) -> (junction 10)
  (junction 10) -> (junction 12) [order 1] : [StallCntOutp >=kMaxStallCnt]
  (junction 10) -> (junction 14) [order 2]
  (junction 12) -> (junction 17)
  (junction 14) -> (junction 17) [order 2]
  (junction 14) -> (junction 16) [order 1] : [SigQlfr<2]
  (junction 17) -> (junction 29) : {
      | SigAvl =0;
      | }
  (junction 16) -> (junction 29) : {
      | SigAvl = 1;
      | }
  data: SigRollgCnt input; SigQlfr input; kMaxStallCnt input; SigAvl output uint8; LstRollgCnt input uint8; LstStallCnt input uint8; StallCntOutp output uint8

== stateflow chart ES228A_HwTqArbn/HwTrqArbn/HwTqArbnPer1/Channel Availability/SigAvlChkRev3 ==
  note: SigAvl
      | False = 0
      | Pass = 1
  note: SigQlfr
      | 0 = No Result
      | 1 = Pass
      | 2 = Fail
  (default) -> (junction 2)
  (junction 2) -> (junction 4) [order 1] : [SigRollgCnt ==LstRollgCnt]
  (junction 4) -> (junction 7) [order 2] : {
      | StallCntOutp = LstStallCnt +1;
      | }
  (junction 2) -> (junction 3) [order 2]
  (junction 4) -> (junction 7) [order 1] : [LstStallCnt == 255]
      | {
      | StallCntOutp = 255;
      | }
  (junction 3) -> (junction 7) : {
      | StallCntOutp = 0;
      | }
  (junction 7) -> (junction 10)
  (junction 10) -> (junction 12) [order 1] : [StallCntOutp >=kMaxStallCnt]
  (junction 10) -> (junction 14) [order 2]
  (junction 12) -> (junction 17)
  (junction 14) -> (junction 17) [order 2]
  (junction 14) -> (junction 16) [order 1] : [SigQlfr<2]
  (junction 17) -> (junction 29) : {
      | SigAvl =0;
      | }
  (junction 16) -> (junction 29) : {
      | SigAvl = 1;
      | }
  data: SigRollgCnt input; SigQlfr input; kMaxStallCnt input; SigAvl output uint8; LstRollgCnt input uint8; LstStallCnt input uint8; StallCntOutp output uint8

== stateflow chart ES228A_HwTqArbn/HwTrqArbn/HwTqArbnPer1/Channel Availability/SigAvlChkRev4 ==
  note: SigAvl
      | False = 0
      | Pass = 1
  note: SigQlfr
      | 0 = No Result
      | 1 = Pass
      | 2 = Fail
  (default) -> (junction 2)
  (junction 2) -> (junction 4) [order 1] : [SigRollgCnt ==LstRollgCnt]
  (junction 4) -> (junction 7) [order 2] : {
      | StallCntOutp = LstStallCnt +1;
      | }
  (junction 2) -> (junction 3) [order 2]
  (junction 4) -> (junction 7) [order 1] : [LstStallCnt == 255]
      | {
      | StallCntOutp = 255;
      | }
  (junction 3) -> (junction 7) : {
      | StallCntOutp = 0;
      | }
  (junction 7) -> (junction 10)
  (junction 10) -> (junction 12) [order 1] : [StallCntOutp >=kMaxStallCnt]
  (junction 10) -> (junction 14) [order 2]
  (junction 12) -> (junction 17)
  (junction 14) -> (junction 17) [order 2]
  (junction 14) -> (junction 16) [order 1] : [SigQlfr<2]
  (junction 17) -> (junction 29) : {
      | SigAvl =0;
      | }
  (junction 16) -> (junction 29) : {
      | SigAvl = 1;
      | }
  data: SigRollgCnt input; SigQlfr input; kMaxStallCnt input; SigAvl output uint8; LstRollgCnt input uint8; LstStallCnt input uint8; StallCntOutp output uint8
